simulink model "aero2vr"  (Simulink 3.00)
settings: Solver=ode45  StartTime=0.0  StopTime=10.0  RelTol=1e-3
libraries: simulink3 x20
settings Model: ExtModeTrigMode=normal  ExtModeArmWhenConnect=on  LastModifiedBy=campa

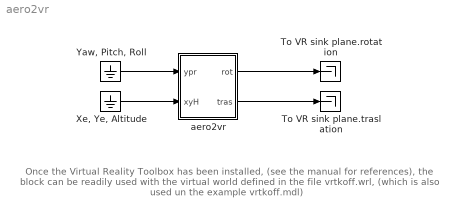
== system aero2vr ==
  note: Once the Virtual Reality Toolbox has been installed,
      | (see the manual for references), the block can be readily
      | used with the virtual world defined in the file vrtkoff.wrl,
      | (which is also used un the example vrtkoff.mdl)
  To VR sink plane.rotation : Terminator
  To VR sink plane.traslation : Terminator
  "Xe, Ye, Altitude" : Ground
  "Yaw, Pitch, Roll" : Ground
  aero2vr : Subsystem
      mask Type: VR Toolbox Interface
      mask Description:
      | Input 1 :    Yaw, Pitch, Roll angles in radians
      |   Input 2 :    X position, Y position, Altitude
      |   Output 1 : Plane.rotation for VR Sink
      |   Output 2 : Plane.translation for VR Sink
      mask Help:
      | <p>
      | The standard aeronautics conventions
      | place on an aircraft a fixed "body
      | reference frame" with the x axis pointing
      | forward, the y axis pointing starboard,
      | and z=cross(x,y) pointing downward.
      | The "earth reference frame" instead is
      | earth-fixed and has the X axis pointing
      | north, the Y axis pointing east, and
      | since Z=cross(X,Y) the Z axis points
      | down towards the earth center.
      | </p>
      | <p>
      | The orientation and position of the body
      | axis with respect to the earth axis is
      | then expressed respectively by means of
      | euler angles (rotation), and cartesian
      | coordinates (translation) X,Y, and H=-Z.
      | </p>
      | <p>
      | For further info on conventions used
      | in aeronautics see for example the FDC
      | Toolbox available in the matlab central.
      | </p>
      | <p>
      | In a VRML virtual world, the "main" axis
      | of the world follow the standard VRML
      | convention, (www.web3d.org/vrml/vrml.htm),
      | and the orientation of a reference frame
      | is expressed by means of the Rodrigues
      | a.k.a. vector-angle, notation formula:
      | R=exp(angle*Skew(vector)).
      | </p>
      | <p>
      | Anyway, mind that any viewpoint is
      | usually defined with its own orientation.
      | For example, in the file wrtkoff.wrl,
      | viewpoint the "ride on the airplane"
      | is such that, facing the monitor,
      | x points to the left,
      | y points above, and z ahead.
      | <p/>
      | <p>
      | This block allows the use of aeronautics
      | conventions to express orientation and
      | position of an object in a virtual world.
      | In other words, the object's orientation
      | can be expressed by means of euler angles
      | and its position by means of X,Y, and H
      | cartesian coordinates.
      | <p/>
      | <p>
      | Specifically, the first and second inputs are
      | the Yaw, Pitch, Roll angles in radians and
      | the X position, Y position, Altitude. <br>
      | The outputs are the vectors "Plane.rotation" and
      | "Plane.translation" for the VR Sink block
      | <p/>
      | <p>
      | Giampiero Campa, WVU, 10/10/02
      | <p/>
  wires:
  aero2vr/1(rot) -> To VR sink plane.rotation/1
  aero2vr/2(tras) -> To VR sink plane.traslation/1
  "Yaw, Pitch, Roll"/1 -> aero2vr/1(ypr)
  "Xe, Ye, Altitude"/1 -> aero2vr/2(xyH)

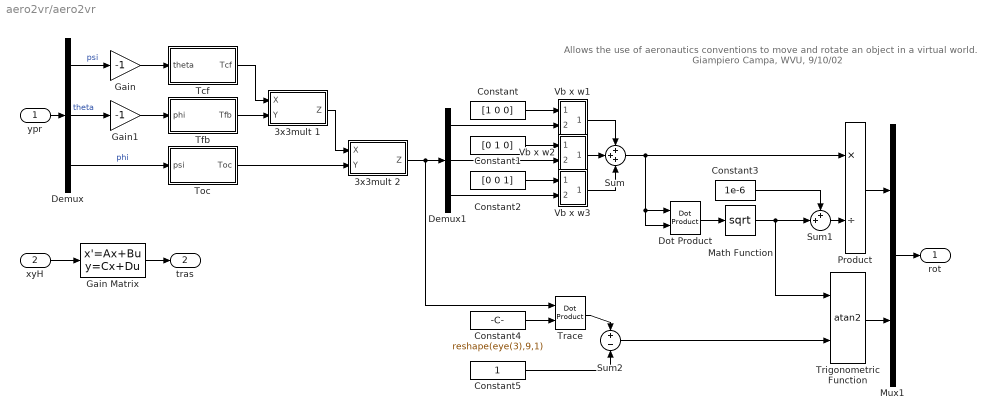
== system aero2vr/aero2vr ==
  note: Allows the use of aeronautics conventions to
      | move and rotate an object in a virtual world.
      | Giampiero Campa, WVU, 9/10/02
  ypr : Inport  Port=1  PortWidth=-1  SampleTime=-1  DataType=auto
      settings: SignalType=auto
  xyH : Inport  Port=2  PortWidth=-1  SampleTime=-1  DataType=auto
      settings: SignalType=auto
  3x3mult 1 : Subsystem
      mask Type: 3x3 Matrix Multiplication
      mask Description:
      | Input 1   : elements of matrix X (3 by 3)
      |   Input 2   : elements of matrix Y (3 by 3)
      |   Output   : elements of matrix X*Y (3 by 3)
      mask Help:
      | <p>
      | Elements of input and output matrices are taken columnwise.
      | </p>
      mask Display: disp('Z=X*Y')
  3x3mult 2 : Subsystem
      mask Type: 3x3 Matrix Multiplication
      mask Description:
      | Input 1   : elements of matrix X (3 by 3)
      |   Input 2   : elements of matrix Y (3 by 3)
      |   Output   : elements of matrix X*Y (3 by 3)
      mask Help:
      | <p>
      | Elements of input and output matrices are taken columnwise.
      | </p>
      mask Display: disp('Z=X*Y')
  Constant : Constant  Value=[1 0 0]
  Constant1 : Constant  Value=[0 1 0]
  Constant2 : Constant  Value=[0 0 1]
  Constant3 : Constant  Value=1e-6
  Constant4 : Constant  Value=reshape(eye(3),9,1)
  Constant5 : Constant  Value=1
  Demux : Demux  Outputs=3
  Demux1 : Demux  Outputs=[3 3 3]
  Dot Product : simulink3/Math/Dot Product
  Gain : Gain  Gain=-1  SaturateOnIntegerOverflow=on
  Gain Matrix : StateSpace  A=[]  B=[]  C=[]  D=[0 -1 0; 0 0 1; 1 0 0]  X0=0
  Gain1 : Gain  Gain=-1  SaturateOnIntegerOverflow=on
  Math Function : Math  Operator=sqrt  OutputSignalType=auto
  Mux1 : Mux  Inputs=2
  Product : Product  Inputs=*/  SaturateOnIntegerOverflow=on
  Sum : Sum  Inputs=+++  SaturateOnIntegerOverflow=on
  Sum1 : Sum  Inputs=++|  SaturateOnIntegerOverflow=on
  Sum2 : Sum  Inputs=+-  SaturateOnIntegerOverflow=on
  Tcf : Subsystem
  Tfb : Subsystem
  Toc : Subsystem
  Trace : simulink3/Math/Dot Product
  Trigonometric Function : Trigonometry  Operator=atan2  OutputSignalType=auto
  Vb x w1 : Subsystem
      mask Type: Cross Product
      mask Description: Calculates the cross product of two 3x1 vectors.
      mask Help:
      | <p>This block calculates the cross product of two 3x1 vectors, ie.</p>
      | 
      | <ul>C(1) = A(2)*B(3) - A(3)*B(2)</ul>
      | <ul>C(2) = A(3)*B(1) - A(1)*B(3)</ul>
      | <ul>C(3) = A(1)*B(2) - A(2)*B(1)</ul>
      | 
      | <p>The block inputs and output contain more than one signal as described below.</p>
      | 
      | <p><H4>Block Vector Input 1 - A</H4>
      | <ul>
      | <li>A(1)</li>
      | <li>A(2)</li>
      | <li>A(3)</li>
      | </ul>
      | </p>
      | 
      | <p><H4>Block Vector Input 2 - B</H4>
      | <ul>
      | <li>B(1)</li>
      | <li>B(2)</li>
      | <li>B(3)</li>
      | </ul>
      | </p>
      | 
      | <p><H4>Block Vector Output - Cross Product (AxB)</H4>
      | <ul>
      | <li>C(1)</li>
      | <li>C(2)</li>
      | <li>C(3)</li>
      | </ul>
      | </p>
      mask Display: disp('Cross\nProduct')
  Vb x w2 : Subsystem
      mask Type: Cross Product
      mask Description: Calculates the cross product of two 3x1 vectors.
      mask Help:
      | <p>This block calculates the cross product of two 3x1 vectors, ie.</p>
      | 
      | <ul>C(1) = A(2)*B(3) - A(3)*B(2)</ul>
      | <ul>C(2) = A(3)*B(1) - A(1)*B(3)</ul>
      | <ul>C(3) = A(1)*B(2) - A(2)*B(1)</ul>
      | 
      | <p>The block inputs and output contain more than one signal as described below.</p>
      | 
      | <p><H4>Block Vector Input 1 - A</H4>
      | <ul>
      | <li>A(1)</li>
      | <li>A(2)</li>
      | <li>A(3)</li>
      | </ul>
      | </p>
      | 
      | <p><H4>Block Vector Input 2 - B</H4>
      | <ul>
      | <li>B(1)</li>
      | <li>B(2)</li>
      | <li>B(3)</li>
      | </ul>
      | </p>
      | 
      | <p><H4>Block Vector Output - Cross Product (AxB)</H4>
      | <ul>
      | <li>C(1)</li>
      | <li>C(2)</li>
      | <li>C(3)</li>
      | </ul>
      | </p>
      mask Display: disp('Cross\nProduct')
  Vb x w3 : Subsystem
      mask Type: Cross Product
      mask Description: Calculates the cross product of two 3x1 vectors.
      mask Help:
      | <p>This block calculates the cross product of two 3x1 vectors, ie.</p>
      | 
      | <ul>C(1) = A(2)*B(3) - A(3)*B(2)</ul>
      | <ul>C(2) = A(3)*B(1) - A(1)*B(3)</ul>
      | <ul>C(3) = A(1)*B(2) - A(2)*B(1)</ul>
      | 
      | <p>The block inputs and output contain more than one signal as described below.</p>
      | 
      | <p><H4>Block Vector Input 1 - A</H4>
      | <ul>
      | <li>A(1)</li>
      | <li>A(2)</li>
      | <li>A(3)</li>
      | </ul>
      | </p>
      | 
      | <p><H4>Block Vector Input 2 - B</H4>
      | <ul>
      | <li>B(1)</li>
      | <li>B(2)</li>
      | <li>B(3)</li>
      | </ul>
      | </p>
      | 
      | <p><H4>Block Vector Output - Cross Product (AxB)</H4>
      | <ul>
      | <li>C(1)</li>
      | <li>C(2)</li>
      | <li>C(3)</li>
      | </ul>
      | </p>
      mask Display: disp('Cross\nProduct')
  rot : Outport  Port=1
  tras : Outport  Port=2
  wires:
  Trace/1 -> Sum2/1
  Mux1/1 -> rot/1
  Demux1/3 -> Vb x w3/2(b(1) b(2) b(3))
  Demux1/1 -> Vb x w1/2(b(1) b(2) b(3))
  Demux1/2 -> Vb x w2/2(b(1) b(2) b(3))
  Toc/1(Toc) -> 3x3mult 2/2(Y)
  Demux/3 -> Toc/1(psi)  "phi"
  Gain1/1 -> Tfb/1(phi)
  Gain/1 -> Tcf/1(theta)
  Demux/2 -> Gain1/1  "theta"
  Tfb/1(Tfb) -> 3x3mult 1/2(Y)
  Tcf/1(Tcf) -> 3x3mult 1/1(X)
  Demux/1 -> Gain/1  "psi"
  Constant5/1 -> Sum2/2
  Sum2/1 -> Trigonometric Function/2
  Constant4/1 -> Trace/2
  Trigonometric Function/1 -> Mux1/2
  Math Function/1 -> Sum1/2, Trigonometric Function/1
  Dot Product/1 -> Math Function/1
  Sum/1 -> Product/1, Dot Product/1, Dot Product/2
  Sum1/1 -> Product/2
  Constant3/1 -> Sum1/1
  Product/1 -> Mux1/1
  Vb x w3/1(c(1) c(2) c(3)) -> Sum/3
  Vb x w2/1(c(1) c(2) c(3)) -> Sum/2
  Vb x w1/1(c(1) c(2) c(3)) -> Sum/1
  Constant2/1 -> Vb x w3/1(a(1) a(2) a(3))
  Constant1/1 -> Vb x w2/1(a(1) a(2) a(3))
  Constant/1 -> Vb x w1/1(a(1) a(2) a(3))
  3x3mult 2/1(Z) -> Trace/1, Demux1/1
  3x3mult 1/1(Z) -> 3x3mult 2/1(X)
  ypr/1 -> Demux/1
  xyH/1 -> Gain Matrix/1
  Gain Matrix/1 -> tras/1

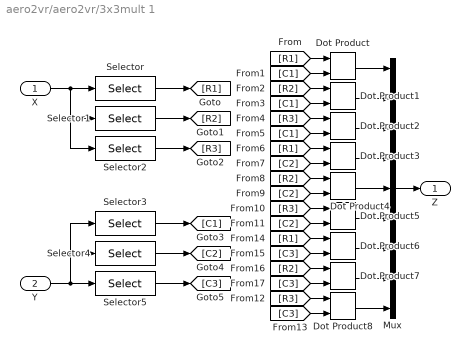
== system aero2vr/aero2vr/3x3mult 1 ==
  X : Inport  Port=1  PortWidth=-1  SampleTime=-1  DataType=auto
      settings: SignalType=auto
  Y : Inport  Port=2  PortWidth=-1  SampleTime=-1  DataType=auto
      settings: SignalType=auto
  Dot Product{,1..8} (9 alike) : simulink3/Math/Dot Product
  Mux : Mux  Inputs=9
  Selector : Selector  Elements=[0 3 6]+1  InputPortWidth=9
  Selector1 : Selector  Elements=[0 3 6]+2  InputPortWidth=9
  Selector2 : Selector  Elements=[0 3 6]+3  InputPortWidth=9
  Selector3 : Selector  Elements=[0 1 2]+1  InputPortWidth=9
  Selector4 : Selector  Elements=[0 1 2]+4  InputPortWidth=9
  Selector5 : Selector  Elements=[0 1 2]+7  InputPortWidth=9
  Z : Outport  Port=1
  wires:
  X/1 -> Selector/1, Selector1/1, Selector2/1
  Selector/1 -> [R1]
  Dot Product/1 -> Mux/1
  Dot Product1/1 -> Mux/2
  Dot Product2/1 -> Mux/3
  [R1] -> Dot Product/1
  [C1] -> Dot Product/2
  [R2] -> Dot Product1/1
  [C1] -> Dot Product1/2
  [R3] -> Dot Product2/1
  [C1] -> Dot Product2/2
  [R1] -> Dot Product3/1
  [C2] -> Dot Product3/2
  [R2] -> Dot Product4/1
  [C2] -> Dot Product4/2
  [R3] -> Dot Product5/1
  [R1] -> Dot Product6/1
  [C3] -> Dot Product6/2
  [R2] -> Dot Product7/1
  [C3] -> Dot Product7/2
  [R3] -> Dot Product8/1
  [C2] -> Dot Product5/2
  [C3] -> Dot Product8/2
  Dot Product3/1 -> Mux/4
  Dot Product4/1 -> Mux/5
  Dot Product5/1 -> Mux/6
  Dot Product6/1 -> Mux/7
  Dot Product7/1 -> Mux/8
  Dot Product8/1 -> Mux/9
  Y/1 -> Selector5/1, Selector4/1, Selector3/1
  Selector5/1 -> [C3]
  Selector1/1 -> [R2]
  Selector2/1 -> [R3]
  Selector4/1 -> [C2]
  Selector3/1 -> [C1]
  Mux/1 -> Z/1

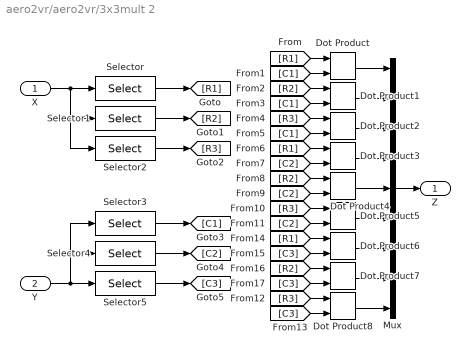
== system aero2vr/aero2vr/3x3mult 2 ==
  X : Inport  Port=1  PortWidth=-1  SampleTime=-1  DataType=auto
      settings: SignalType=auto
  Y : Inport  Port=2  PortWidth=-1  SampleTime=-1  DataType=auto
      settings: SignalType=auto
  Dot Product{,1..8} (9 alike) : simulink3/Math/Dot Product
  Mux : Mux  Inputs=9
  Selector : Selector  Elements=[0 3 6]+1  InputPortWidth=9
  Selector1 : Selector  Elements=[0 3 6]+2  InputPortWidth=9
  Selector2 : Selector  Elements=[0 3 6]+3  InputPortWidth=9
  Selector3 : Selector  Elements=[0 1 2]+1  InputPortWidth=9
  Selector4 : Selector  Elements=[0 1 2]+4  InputPortWidth=9
  Selector5 : Selector  Elements=[0 1 2]+7  InputPortWidth=9
  Z : Outport  Port=1
  wires:
  Mux/1 -> Z/1
  Selector3/1 -> [C1]
  Selector4/1 -> [C2]
  Selector2/1 -> [R3]
  Selector1/1 -> [R2]
  Selector5/1 -> [C3]
  Y/1 -> Selector3/1, Selector4/1, Selector5/1
  Dot Product8/1 -> Mux/9
  Dot Product7/1 -> Mux/8
  Dot Product6/1 -> Mux/7
  Dot Product5/1 -> Mux/6
  Dot Product4/1 -> Mux/5
  Dot Product3/1 -> Mux/4
  [C3] -> Dot Product8/2
  [C2] -> Dot Product5/2
  [R3] -> Dot Product8/1
  [C3] -> Dot Product7/2
  [R2] -> Dot Product7/1
  [C3] -> Dot Product6/2
  [R1] -> Dot Product6/1
  [R3] -> Dot Product5/1
  [C2] -> Dot Product4/2
  [R2] -> Dot Product4/1
  [C2] -> Dot Product3/2
  [R1] -> Dot Product3/1
  [C1] -> Dot Product2/2
  [R3] -> Dot Product2/1
  [C1] -> Dot Product1/2
  [R2] -> Dot Product1/1
  [C1] -> Dot Product/2
  [R1] -> Dot Product/1
  Dot Product2/1 -> Mux/3
  Dot Product1/1 -> Mux/2
  Dot Product/1 -> Mux/1
  Selector/1 -> [R1]
  X/1 -> Selector2/1, Selector1/1, Selector/1

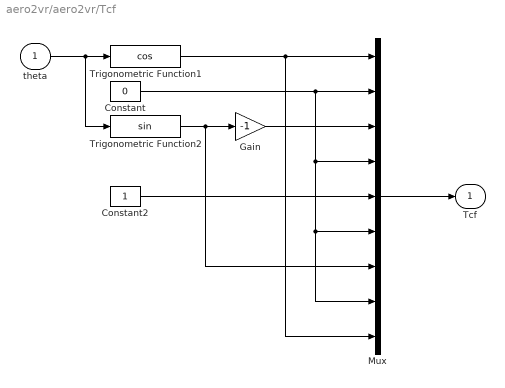
== system aero2vr/aero2vr/Tcf ==
  theta : Inport  Port=1  PortWidth=-1  SampleTime=-1  DataType=auto
      settings: SignalType=auto
  Constant : Constant  Value=0
  Constant2 : Constant  Value=1
  Gain : Gain  Gain=-1  SaturateOnIntegerOverflow=on
  Mux : Mux  Inputs=9
  Trigonometric Function1 : Trigonometry  Operator=cos  OutputSignalType=auto
  Trigonometric Function2 : Trigonometry  Operator=sin  OutputSignalType=auto
  Tcf : Outport  Port=1
  wires:
  Mux/1 -> Tcf/1
  theta/1 -> Trigonometric Function2/1, Trigonometric Function1/1
  Gain/1 -> Mux/3
  Constant/1 -> Mux/2, Mux/4, Mux/6, Mux/8
  Constant2/1 -> Mux/5
  Trigonometric Function2/1 -> Gain/1, Mux/7
  Trigonometric Function1/1 -> Mux/1, Mux/9

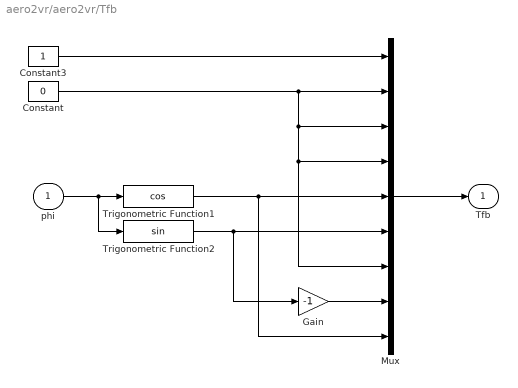
== system aero2vr/aero2vr/Tfb ==
  phi : Inport  Port=1  PortWidth=-1  SampleTime=-1  DataType=auto
      settings: SignalType=auto
  Constant : Constant  Value=0
  Constant3 : Constant  Value=1
  Gain : Gain  Gain=-1  SaturateOnIntegerOverflow=on
  Mux : Mux  Inputs=9
  Trigonometric Function1 : Trigonometry  Operator=cos  OutputSignalType=auto
  Trigonometric Function2 : Trigonometry  Operator=sin  OutputSignalType=auto
  Tfb : Outport  Port=1
  wires:
  Mux/1 -> Tfb/1
  Constant3/1 -> Mux/1
  Constant/1 -> Mux/2, Mux/3, Mux/4, Mux/7
  phi/1 -> Trigonometric Function1/1, Trigonometric Function2/1
  Trigonometric Function2/1 -> Mux/6, Gain/1
  Gain/1 -> Mux/8
  Trigonometric Function1/1 -> Mux/5, Mux/9

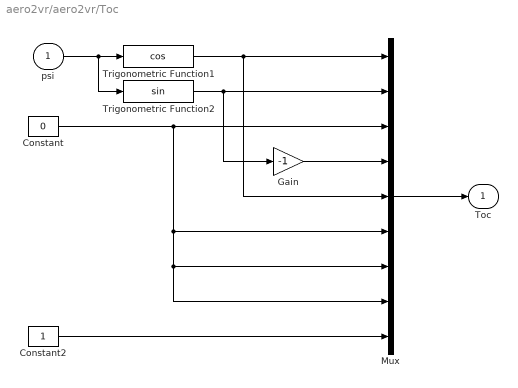
== system aero2vr/aero2vr/Toc ==
  psi : Inport  Port=1  PortWidth=-1  SampleTime=-1  DataType=auto
      settings: SignalType=auto
  Constant : Constant  Value=0
  Constant2 : Constant  Value=1
  Gain : Gain  Gain=-1  SaturateOnIntegerOverflow=on
  Mux : Mux  Inputs=9
  Trigonometric Function1 : Trigonometry  Operator=cos  OutputSignalType=auto
  Trigonometric Function2 : Trigonometry  Operator=sin  OutputSignalType=auto
  Toc : Outport  Port=1
  wires:
  psi/1 -> Trigonometric Function1/1, Trigonometric Function2/1
  Trigonometric Function1/1 -> Mux/1, Mux/5
  Trigonometric Function2/1 -> Gain/1, Mux/2
  Gain/1 -> Mux/4
  Constant2/1 -> Mux/9
  Constant/1 -> Mux/3, Mux/7, Mux/8, Mux/6
  Mux/1 -> Toc/1

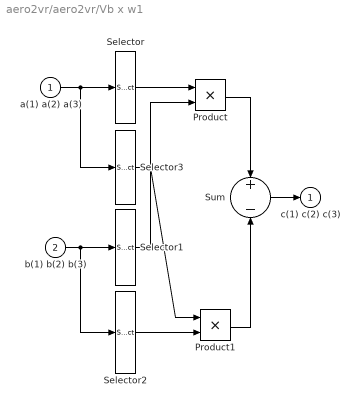
== system aero2vr/aero2vr/Vb x w1 ==
  a(1) a(2) a(3) : Inport  Port=1  PortWidth=-1  SampleTime=-1  DataType=auto
      settings: SignalType=auto
  b(1) b(2) b(3) : Inport  Port=2  PortWidth=-1  SampleTime=-1  DataType=auto
      settings: SignalType=auto
  Product : Product  Inputs=2  SaturateOnIntegerOverflow=on
  Product1 : Product  Inputs=2  SaturateOnIntegerOverflow=on
  Selector : Selector  Elements=[2 3 1]  InputPortWidth=3
  Selector1 : Selector  Elements=[3 1 2]  InputPortWidth=3
  Selector2 : Selector  Elements=[2 3 1]  InputPortWidth=3
  Selector3 : Selector  Elements=[3 1 2]  InputPortWidth=3
  Sum : Sum  Inputs=+|-  SaturateOnIntegerOverflow=on
  c(1) c(2) c(3) : Outport  Port=1  InitialOutput=0
  wires:
  Sum/1 -> c(1) c(2) c(3)/1
  b(1) b(2) b(3)/1 -> Selector1/1, Selector2/1
  Selector/1 -> Product/1
  a(1) a(2) a(3)/1 -> Selector/1, Selector3/1
  Product/1 -> Sum/1
  Selector1/1 -> Product/2
  Product1/1 -> Sum/2
  Selector2/1 -> Product1/2
  Selector3/1 -> Product1/1

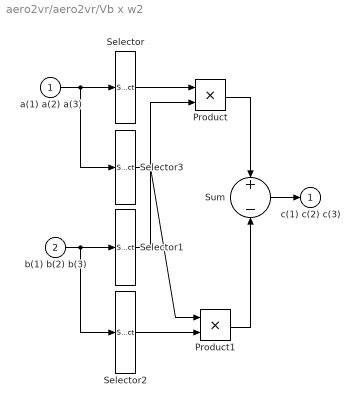
== system aero2vr/aero2vr/Vb x w2 ==
  a(1) a(2) a(3) : Inport  Port=1  PortWidth=-1  SampleTime=-1  DataType=auto
      settings: SignalType=auto
  b(1) b(2) b(3) : Inport  Port=2  PortWidth=-1  SampleTime=-1  DataType=auto
      settings: SignalType=auto
  Product : Product  Inputs=2  SaturateOnIntegerOverflow=on
  Product1 : Product  Inputs=2  SaturateOnIntegerOverflow=on
  Selector : Selector  Elements=[2 3 1]  InputPortWidth=3
  Selector1 : Selector  Elements=[3 1 2]  InputPortWidth=3
  Selector2 : Selector  Elements=[2 3 1]  InputPortWidth=3
  Selector3 : Selector  Elements=[3 1 2]  InputPortWidth=3
  Sum : Sum  Inputs=+|-  SaturateOnIntegerOverflow=on
  c(1) c(2) c(3) : Outport  Port=1  InitialOutput=0
  wires:
  Sum/1 -> c(1) c(2) c(3)/1
  b(1) b(2) b(3)/1 -> Selector1/1, Selector2/1
  Selector/1 -> Product/1
  a(1) a(2) a(3)/1 -> Selector/1, Selector3/1
  Product/1 -> Sum/1
  Selector1/1 -> Product/2
  Product1/1 -> Sum/2
  Selector2/1 -> Product1/2
  Selector3/1 -> Product1/1

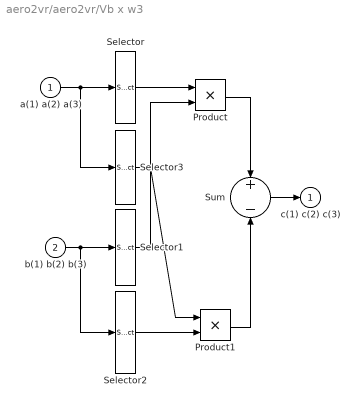
== system aero2vr/aero2vr/Vb x w3 ==
  a(1) a(2) a(3) : Inport  Port=1  PortWidth=-1  SampleTime=-1  DataType=auto
      settings: SignalType=auto
  b(1) b(2) b(3) : Inport  Port=2  PortWidth=-1  SampleTime=-1  DataType=auto
      settings: SignalType=auto
  Product : Product  Inputs=2  SaturateOnIntegerOverflow=on
  Product1 : Product  Inputs=2  SaturateOnIntegerOverflow=on
  Selector : Selector  Elements=[2 3 1]  InputPortWidth=3
  Selector1 : Selector  Elements=[3 1 2]  InputPortWidth=3
  Selector2 : Selector  Elements=[2 3 1]  InputPortWidth=3
  Selector3 : Selector  Elements=[3 1 2]  InputPortWidth=3
  Sum : Sum  Inputs=+|-  SaturateOnIntegerOverflow=on
  c(1) c(2) c(3) : Outport  Port=1  InitialOutput=0
  wires:
  Sum/1 -> c(1) c(2) c(3)/1
  b(1) b(2) b(3)/1 -> Selector1/1, Selector2/1
  Selector/1 -> Product/1
  a(1) a(2) a(3)/1 -> Selector/1, Selector3/1
  Product/1 -> Sum/1
  Selector1/1 -> Product/2
  Product1/1 -> Sum/2
  Selector2/1 -> Product1/2
  Selector3/1 -> Product1/1
